simulink model "ResonantSystem"  (R2023b)
settings: Solver=VariableStepAuto  StartTime=0.0  StopTime=20  RelTol=1e-3
values from neighbouring files (symbols this model uses):
  G5_den = [a,b,c,d,e,f,g,h]    [ResonantSystem_ElectricalFilterWithMultiplePoles.m]
  G5_num = [A,B,C,D,E,F,G]    [ResonantSystem_ElectricalFilterWithMultiplePoles.m]
settings Model: Creator=Sofia Katrina Dilag  LastModifiedBy=Sofia Katrina Dilag

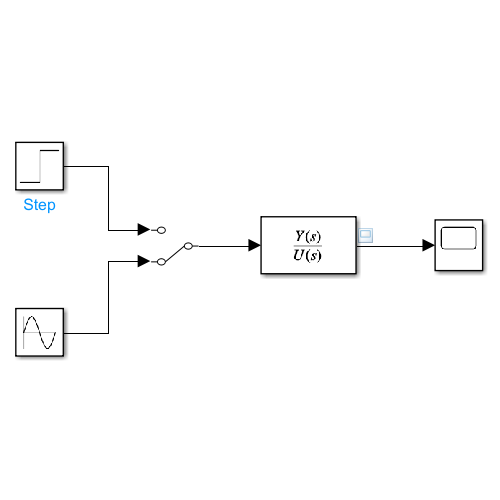
[thumbnail: Simulink's stored preview of the top-level diagram]
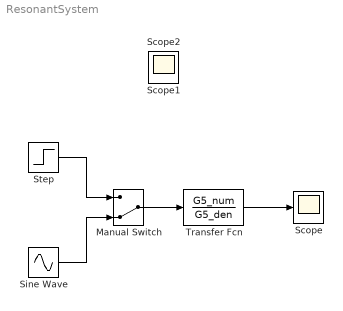
== system ResonantSystem ==
  Manual Switch : ManualSwitch  CurrentSetting=0
  Scope : Scope
  Sine Wave : Sin  SampleTime=0
  Step : Step  Time=0  Before=0.1  SampleTime=0
  Transfer Fcn : TransferFcn  Numerator=G5_num  Denominator=G5_den
  Scope1 : Scope
  Scope2 : Scope
  wires:
  Transfer Fcn/1 -> Scope/1
  Step/1 -> Manual Switch/1
  Sine Wave/1 -> Manual Switch/2
  Manual Switch/1 -> Transfer Fcn/1
